simulink model "sampleModel264"  (R2021b)
settings: Solver=VariableStepAuto  StartTime=0.0  StopTime=10.0  RelTol=1e-3
undefined symbols (not defined in the file or in its folder): DiscIntNeverNeededParam
libraries: simulink x3, slpidlib x2
settings Model: Creator=user  LastModifiedBy=user

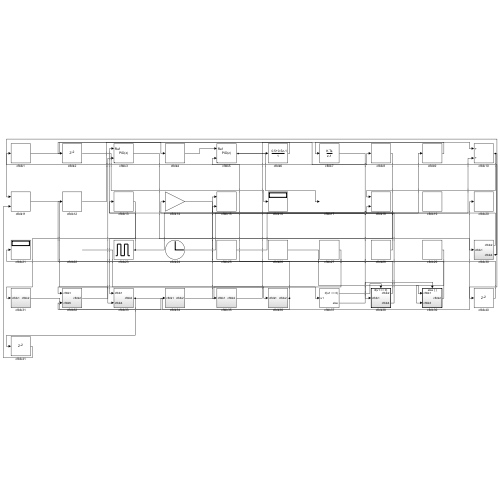
[thumbnail: Simulink's stored preview of the top-level diagram]
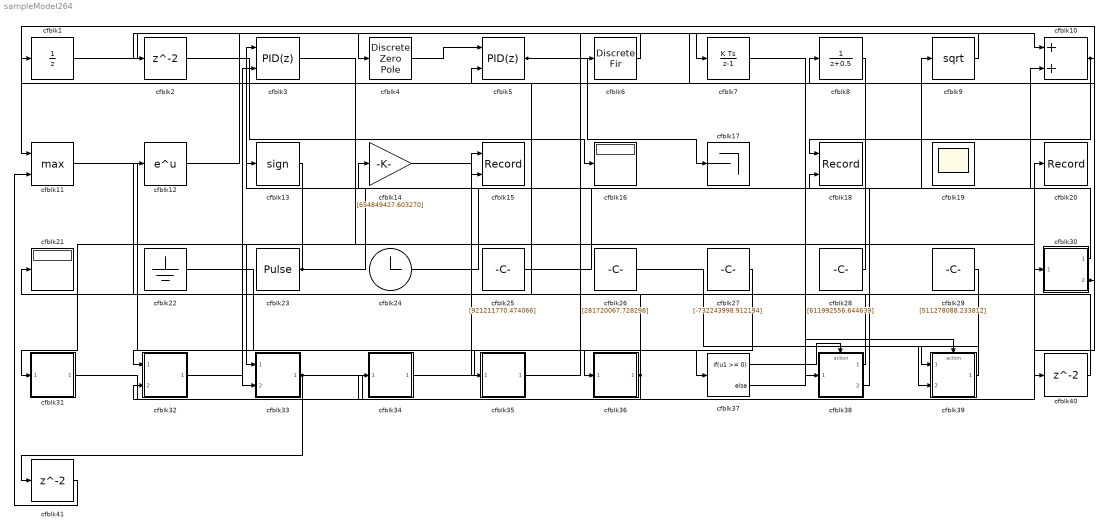
== system sampleModel264 ==
  cfblk1 : UnitDelay  HasFrameUpgradeWarning=on
  cfblk10 : Sum
  cfblk11 : MinMax  Function=max  Inputs=2
  cfblk12 : Math  SaturateOnIntegerOverflow=on
  cfblk13 : Signum
  cfblk14 : Gain  Gain=[654849427.603270]
  cfblk15 : Record  FileSettingsInternal="{\"entries\":[{\"content\":{\"excelSettings\":{\"content\":{},\"type\":\"Streamout.ExcelSettings\"}},\"type\":\"Streamout.FileSettingStorage\",\"uuid\":\"87b09053-a77a-4a9e-8bec-8608d5d060ef\"}],\"packageUris\":[\"http://schema.mathworks.com/mf0/streamout_blocks/R2020a\"],\"version\":\"1.0\"}"  Layout=[1 1]  SignalsInternal="{\"entries\":[{\"content\":{\"signals\":[{\"content\":{\"blockPath\":[\"sampleModel264/cfblk15\"],\"channel\":[],\"dimensions\":[1],\"domain\":\"sampleModel264/cfblk15\",\"lineColor\":\"#a2142f\",\"plots\":[1],\"port\":1,\"sid\":[\"\"],\"signalID\":10963,\"signalName\":\"cfblk38:1\"},\"type\":\"RecordBlkView.Signal\",\"uuid\":\"1c1d3461-8ecc-4c0c-aa7a-5d9b7c4e959a\"},{\"content\":{\"blockPath\":[\"sampleModel264/cfblk15\"],\"channel\":[],\"dimensions\":[1],\"domain\":\"sampleModel264/cfblk15\",\"lineColor\":\"#139fff\",\"plots\":[1],\"port\":2,\"sid\":[\"\"],\"signalID\":10967,\"signalName\":\"cfblk30:1\"},\"type\":\"RecordBlkView.Signal\",\"uuid\":\"7ac7cff1-7016-4733-9738-e051f763ac4b\"}]},\"type\":\"RecordBlkView.InputSignals\",\"uuid\":\"cdef2423-249f-4fef-a01c-88f3f527eae3\"}],\"packageUris\":[\"http://schema.mathworks.com/mf0/streamout_blocks/R2020a\"],\"version\":\"1.0\"}"  VisualizationBindings="{\"xyplotplugin\":{\"info\":[{\"series\":[{\"bindingParametersList\":[{\"parameter\":\"X-Axis\",\"signalID\":10963,\"signalName\":\"cfblk38:1\"},{\"parameter\":\"Y-Axis\",\"signalID\":10967,\"signalName\":\"cfblk30:1\"}],\"seriesID\":8609}],\"subplotID\":1}]}}"  CompatibilityTag=XY
  cfblk16 : Display
  cfblk17 : Terminator
  cfblk18 : Record  FileSettingsInternal="{\"entries\":[{\"content\":{\"excelSettings\":{\"content\":{},\"type\":\"Streamout.ExcelSettings\"}},\"type\":\"Streamout.FileSettingStorage\",\"uuid\":\"e408a021-66fe-4499-80ff-48ba78554e90\"}],\"packageUris\":[\"http://schema.mathworks.com/mf0/streamout_blocks/R2020a\"],\"version\":\"1.0\"}"  Layout=[1 1]  SignalsInternal="{\"entries\":[{\"content\":{\"signals\":[{\"content\":{\"blockPath\":[\"sampleModel264/cfblk18\"],\"channel\":[],\"dimensions\":[1],\"domain\":\"sampleModel264/cfblk18\",\"lineColor\":\"#a2142f\",\"plots\":[1],\"port\":1,\"sid\":[\"\"],\"signalID\":10971,\"signalName\":\"cfblk10\"},\"type\":\"RecordBlkView.Signal\",\"uuid\":\"3a710b1b-58d1-44e6-873a-359d775209f8\"},{\"content\":{\"blockPath\":[\"sampleModel264/cfblk18\"],\"channel\":[],\"dimensions\":[1],\"domain\":\"sampleModel264/cfblk18\",\"lineColor\":\"#139fff\",\"plots\":[1],\"port\":2,\"sid\":[\"\"],\"signalID\":10975,\"signalName\":\"cfblk25\"},\"type\":\"RecordBlkView.Signal\",\"uuid\":\"b2371862-496e-4d84-a68e-603eda18343e\"}]},\"type\":\"RecordBlkView.InputSignals\",\"uuid\":\"b556cba2-bf7e-48f4-b2b5-74105ca156f6\"}],\"packageUris\":[\"http://schema.mathworks.com/mf0/streamout_blocks/R2020a\"],\"version\":\"1.0\"}"  VisualizationBindings="{\"xyplotplugin\":{\"info\":[{\"series\":[{\"bindingParametersList\":[{\"parameter\":\"X-Axis\",\"signalID\":10971,\"signalName\":\"cfblk10\"},{\"parameter\":\"Y-Axis\",\"signalID\":10975,\"signalName\":\"cfblk25\"}],\"seriesID\":10129}],\"subplotID\":1}]}}"  CompatibilityTag=XY
  cfblk19 : Scope
      settings: Floating=on
  cfblk2 : Delay  SampleTime=1
  cfblk20 : Record  FileSettingsInternal="{\"entries\":[{\"content\":{\"excelSettings\":{\"content\":{},\"type\":\"Streamout.ExcelSettings\"}},\"type\":\"Streamout.FileSettingStorage\",\"uuid\":\"be7c116d-fe5e-441c-a5bb-7647be8af16f\"}],\"packageUris\":[\"http://schema.mathworks.com/mf0/streamout_blocks/R2020a\"],\"version\":\"1.0\"}"  SignalsInternal="{\"entries\":[{\"content\":{\"signals\":[{\"content\":{\"blockPath\":[\"sampleModel264/cfblk20\"],\"channel\":[],\"dimensions\":[1],\"domain\":\"sampleModel264/cfblk20\",\"lineColor\":\"#ff6929\",\"plots\":[1],\"port\":1,\"sid\":[\"\"],\"signalID\":10979,\"signalName\":\"cfblk33\"},\"type\":\"RecordBlkView.Signal\",\"uuid\":\"b8781fc3-0edb-411b-9528-19bbc625d2f5\"}]},\"type\":\"RecordBlkView.InputSignals\",\"uuid\":\"c04048e7-6647-4468-bb8a-5f250a700c8b\"}],\"packageUris\":[\"http://schema.mathworks.com/mf0/streamout_blocks/R2020a\"],\"version\":\"1.0\"}"  VisualizationBindings="{\"sparklinesplugin\":{\"info\":[{\"bindingParametersList\":[],\"subplotID\":1}]}}"
  cfblk21 : Display
  cfblk22 : Ground
  cfblk23 : DiscretePulseGenerator  PulseType=Time based  Amplitude=[-625805775.989914]  Period=[26020905.178933]  PulseWidth=5  PhaseDelay=[3.000000]
  cfblk24 : Clock
  cfblk25 : Constant  Value=[921211770.474066]  SampleTime=1
  cfblk26 : Constant  Value=[281720067.728298]  SampleTime=1
  cfblk27 : Constant  Value=[-732243998.912194]  SampleTime=1
  cfblk28 : Constant  Value=[611992556.644639]  SampleTime=1
  cfblk29 : Constant  Value=[511278088.233812]  SampleTime=1
  cfblk3 : slpidlib/PID Controller (2DOF)  Controller=PID  Form=Parallel  TimeDomain=Discrete-time  UseExternalTs=off  SampleTime=1  IntegratorMethod=Forward Euler  FilterMethod=Forward Euler  ControllerParametersSource=internal  P=1  I=1  D=0  UseFilter=on  N=100  b=1  c=1  TunerSelectOption=Transfer Function Based (PID Tuner App)  InitialConditionSource=internal  InitialConditionForIntegrator=0  InitialConditionForFilter=0  DifferentiatorICPrevScaledInput=0  ExternalReset=none  TrackingMode=off  Kt=1  LimitOutput=off  SatLimitsSource=internal  UpperSaturationLimit=inf  LowerSaturationLimit=-inf  LinearizeAsGain=off  AntiWindupMode=none  Kb=1  POutMin=[]  POutMax=[]  IOutMin=[]  IOutMax=[]  DOutMin=[]  DOutMax=[]  NOutMin=[]  NOutMax=[]  bOutMin=[]  bOutMax=[]  cOutMin=[]  cOutMax=[]  SumOutMin=[]  SumOutMax=[]  SaturationOutMin=[]  SaturationOutMax=[]  PParamMin=[]  PParamMax=[]  IParamMin=[]  IParamMax=[]  DParamMin=[]  DParamMax=[]  NParamMin=[]  NParamMax=[]  bParamMin=[]  bParamMax=[]  cParamMin=[]  cParamMax=[]  KbParamMin=[]  KbParamMax=[]  KtParamMin=[]  KtParamMax=[]  KbOutMin=[]  KbOutMax=[]  KtOutMin=[]  KtOutMax=[]  IntegratorOutMin=[]  IntegratorOutMax=[]  FilterOutMin=[]  FilterOutMax=[]  SumI1OutMin=[]  SumI1OutMax=[]  SumI2OutMin=[]  SumI2OutMax=[]  SumI3OutMin=[]  SumI3OutMax=[]  SumI4OutMin=[]  SumI4OutMax=[]  SumDOutMin=[]  SumDOutMax=[]  Sum1OutMin=[]  Sum1OutMax=[]  Sum2OutMin=[]  Sum2OutMax=[]  Sum3OutMin=[]  Sum3OutMax=[]  DifferentiatorOutMin=[]  DifferentiatorOutMax=[]  FilterDiffOutCoefMin=[]  FilterDiffOutCoefMax=[]  ReciprocalOutMin=[]  ReciprocalOutMax=[]  SumDenOutMin=[]  SumDenOutMax=[]  SumNumOutMin=[]  SumNumOutMax=[]  DivideOutMin=[]  DivideOutMax=[]  UdiffTsProdOutMin=[]  UdiffTsProdOutMax=[]  NTsProdOutMin=[]  NTsProdOutMax=[]  UintegralTsProdOutMin=[]  UintegralTsProdOutMax=[]  UngainTsProdOutMin=[]  UngainTsProdOutMax=[]  IntegratorContinuousStateAttributes=''  IntegratorStateMustResolveToSignalObject=off  IntegratorRTWStateStorageClass=Auto  FilterContinuousStateAttributes=''  FilterStateMustResolveToSignalObject=off  FilterRTWStateStorageClass=Auto  ParallelPVariant=InternalParameters  IdealPVariant=Disabled  IVariant=InternalParameters  DVariant=InternalParameters  bVariant=InternalParameters  cVariant=InternalParameters  IntegratorVariant=Discrete  SatVariant=Disabled  AWVariant=Passthrough  PCopyVariant=Disabled  TRVariant=Disabled  FdbkBlocksVariant=Forward  IdealPFdbkVariant=Disabled  SatFdbkVariant=Disabled  DerivativeFilterVariant=ForwardEulerFilter  NVariant=InternalParameters  NCopyVariant=Disabled  FilterICVariant=InternalICsFilter  IntegratorICVariant=InternalICs  ExternalResetVariant=Disabled  TRSumVariant=Passthrough  SumFdbkVariant=Disabled  SumVariant=Sum_PID  TsampFilterVariant=InternalTs  TsampNgainVariant=Passthrough  TsampIntegralVariant=Passthrough  ExternalSaturationOutDataTypeStr=Inherit: Same as second input
      settings: SourceProductBaseCode=SL
  cfblk30 : Subsystem
  cfblk31 : Subsystem
  cfblk32 : Subsystem
  cfblk33 : Subsystem
  cfblk34 : Subsystem
  cfblk35 : Subsystem
  cfblk36 : Subsystem
  cfblk37 : If  IfExpression=u1 >= 0  SampleTime=1
  cfblk38 : Subsystem  TreatAsAtomicUnit=on
  cfblk39 : Subsystem  TreatAsAtomicUnit=on
  cfblk4 : DiscreteZeroPole  Poles=[0 0.5]  Gain=1
  cfblk40 : Delay  SampleTime=1
  cfblk41 : Delay  SampleTime=1
  cfblk5 : slpidlib/PID Controller (2DOF)  Controller=PID  Form=Parallel  TimeDomain=Discrete-time  UseExternalTs=off  SampleTime=1  IntegratorMethod=Forward Euler  FilterMethod=Forward Euler  ControllerParametersSource=internal  P=1  I=1  D=0  UseFilter=on  N=100  b=1  c=1  TunerSelectOption=Transfer Function Based (PID Tuner App)  InitialConditionSource=internal  InitialConditionForIntegrator=0  InitialConditionForFilter=0  DifferentiatorICPrevScaledInput=0  ExternalReset=none  TrackingMode=off  Kt=1  LimitOutput=off  SatLimitsSource=internal  UpperSaturationLimit=inf  LowerSaturationLimit=-inf  LinearizeAsGain=off  AntiWindupMode=none  Kb=1  POutMin=[]  POutMax=[]  IOutMin=[]  IOutMax=[]  DOutMin=[]  DOutMax=[]  NOutMin=[]  NOutMax=[]  bOutMin=[]  bOutMax=[]  cOutMin=[]  cOutMax=[]  SumOutMin=[]  SumOutMax=[]  SaturationOutMin=[]  SaturationOutMax=[]  PParamMin=[]  PParamMax=[]  IParamMin=[]  IParamMax=[]  DParamMin=[]  DParamMax=[]  NParamMin=[]  NParamMax=[]  bParamMin=[]  bParamMax=[]  cParamMin=[]  cParamMax=[]  KbParamMin=[]  KbParamMax=[]  KtParamMin=[]  KtParamMax=[]  KbOutMin=[]  KbOutMax=[]  KtOutMin=[]  KtOutMax=[]  IntegratorOutMin=[]  IntegratorOutMax=[]  FilterOutMin=[]  FilterOutMax=[]  SumI1OutMin=[]  SumI1OutMax=[]  SumI2OutMin=[]  SumI2OutMax=[]  SumI3OutMin=[]  SumI3OutMax=[]  SumI4OutMin=[]  SumI4OutMax=[]  SumDOutMin=[]  SumDOutMax=[]  Sum1OutMin=[]  Sum1OutMax=[]  Sum2OutMin=[]  Sum2OutMax=[]  Sum3OutMin=[]  Sum3OutMax=[]  DifferentiatorOutMin=[]  DifferentiatorOutMax=[]  FilterDiffOutCoefMin=[]  FilterDiffOutCoefMax=[]  ReciprocalOutMin=[]  ReciprocalOutMax=[]  SumDenOutMin=[]  SumDenOutMax=[]  SumNumOutMin=[]  SumNumOutMax=[]  DivideOutMin=[]  DivideOutMax=[]  UdiffTsProdOutMin=[]  UdiffTsProdOutMax=[]  NTsProdOutMin=[]  NTsProdOutMax=[]  UintegralTsProdOutMin=[]  UintegralTsProdOutMax=[]  UngainTsProdOutMin=[]  UngainTsProdOutMax=[]  IntegratorContinuousStateAttributes=''  IntegratorStateMustResolveToSignalObject=off  IntegratorRTWStateStorageClass=Auto  FilterContinuousStateAttributes=''  FilterStateMustResolveToSignalObject=off  FilterRTWStateStorageClass=Auto  ParallelPVariant=InternalParameters  IdealPVariant=Disabled  IVariant=InternalParameters  DVariant=InternalParameters  bVariant=InternalParameters  cVariant=InternalParameters  IntegratorVariant=Discrete  SatVariant=Disabled  AWVariant=Passthrough  PCopyVariant=Disabled  TRVariant=Disabled  FdbkBlocksVariant=Forward  IdealPFdbkVariant=Disabled  SatFdbkVariant=Disabled  DerivativeFilterVariant=ForwardEulerFilter  NVariant=InternalParameters  NCopyVariant=Disabled  FilterICVariant=InternalICsFilter  IntegratorICVariant=InternalICs  ExternalResetVariant=Disabled  TRSumVariant=Passthrough  SumFdbkVariant=Disabled  SumVariant=Sum_PID  TsampFilterVariant=InternalTs  TsampNgainVariant=Passthrough  TsampIntegralVariant=Passthrough  ExternalSaturationOutDataTypeStr=Inherit: Same as second input
      settings: SourceProductBaseCode=SL
  cfblk6 : DiscreteFir  SampleTime=1
  cfblk7 : DiscreteIntegrator  ICPrevOutput=DiscIntNeverNeededParam  ICPrevScaledInput=DiscIntNeverNeededParam
  cfblk8 : DiscreteTransferFcn  SampleTime=1
  cfblk9 : Sqrt  SaturateOnIntegerOverflow=on
  wires:
  cfblk5/1 -> cfblk17/1, cfblk10/1
  cfblk23/1 -> cfblk3/1, cfblk10/2
  cfblk9/1 -> cfblk7/1
  cfblk12/1 -> cfblk8/1
  cfblk1/1 -> cfblk4/1
  cfblk2/1 -> cfblk16/1
  cfblk36/1(cfblk2) -> cfblk21/1, cfblk32/2(cfblk5)
  cfblk33/1(cfblk2) -> cfblk20/1, cfblk41/1
  cfblk34/1(cfblk2) -> cfblk37/1
  cfblk13/1 -> cfblk31/1(cfblk1)
  cfblk8/1 -> cfblk33/1(cfblk1)
  cfblk22/1 -> cfblk36/1(cfblk1)
  cfblk26/1 -> cfblk39/1(cfblk1)
  cfblk35/1(cfblk2) -> cfblk6/1
  cfblk31/1(cfblk2) -> cfblk34/1(cfblk1)
  cfblk32/1(cfblk2) -> cfblk3/2
  cfblk11/1 -> cfblk33/2(cfblk4)
  cfblk38/1(cfblk2) -> cfblk15/1
  cfblk28/1 -> cfblk13/1
  cfblk14/1 -> cfblk35/1(cfblk1)
  cfblk39/1(cfblk2) -> cfblk12/1
  cfblk3/1 -> cfblk30/1(cfblk1)
  cfblk29/1 -> cfblk39/2(cfblk3)
  cfblk38/2(cfblk4) -> cfblk14/1
  cfblk6/1 -> cfblk2/1
  cfblk24/1 -> cfblk9/1
  cfblk30/1(cfblk2) -> cfblk15/2
  cfblk30/2(cfblk4) -> cfblk11/1, cfblk1/1
  cfblk7/1 -> cfblk38/1(cfblk1)
  cfblk10/1 -> cfblk18/1, cfblk40/1
  cfblk4/1 -> cfblk5/1
  cfblk27/1 -> cfblk32/1(cfblk1)
  cfblk25/1 -> cfblk18/2
  cfblk37/1 -> cfblk38/Action
  cfblk37/2 -> cfblk39/Action
  cfblk40/1 -> cfblk5/2
  cfblk41/1 -> cfblk11/2

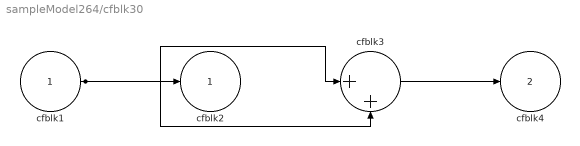
== system sampleModel264/cfblk30 ==
  cfblk1 : Inport
  cfblk3 : Sum  Inputs=|++
  cfblk2 : Outport
  cfblk4 : Outport  Port=2
  wires:
  cfblk3/1 -> cfblk4/1
  cfblk1/1 -> cfblk2/1, cfblk3/1, cfblk3/2

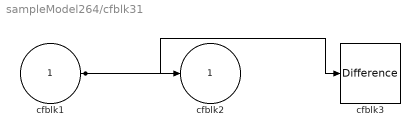
== system sampleModel264/cfblk31 ==
  cfblk1 : Inport
  cfblk3 : simulink/Discrete/Difference  ICPrevInput=0.0  OutMin=[]  OutMax=[]  OutDataTypeStr=Inherit: Inherit via back propagation  OutDataType=fixdt(1, 16)  OutScaling=2^-10  DoSatur=off
  cfblk2 : Outport
  wires:
  cfblk1/1 -> cfblk2/1, cfblk3/1

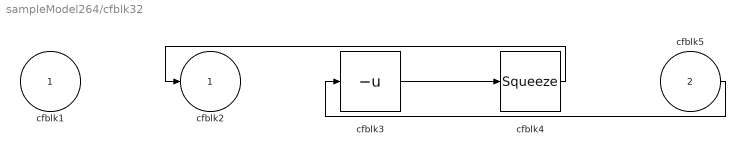
== system sampleModel264/cfblk32 ==
  cfblk1 : Inport
  cfblk5 : Inport  Port=2
  cfblk3 : UnaryMinus
  cfblk4 : Squeeze
  cfblk2 : Outport
  wires:
  cfblk4/1 -> cfblk2/1
  cfblk5/1 -> cfblk3/1
  cfblk3/1 -> cfblk4/1

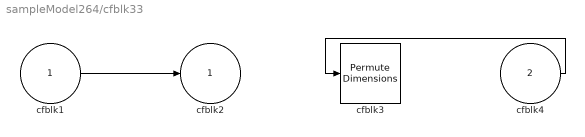
== system sampleModel264/cfblk33 ==
  cfblk1 : Inport
  cfblk4 : Inport  Port=2
  cfblk3 : PermuteDimensions
  cfblk2 : Outport
  wires:
  cfblk4/1 -> cfblk3/1
  cfblk1/1 -> cfblk2/1

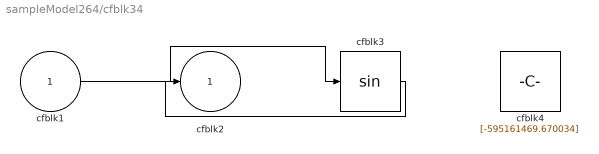
== system sampleModel264/cfblk34 ==
  cfblk1 : Inport
  cfblk3 : Trigonometry
  cfblk4 : Constant  Value=[-595161469.670034]  SampleTime=1
  cfblk2 : Outport
  wires:
  cfblk1/1 -> cfblk3/1
  cfblk3/1 -> cfblk2/1

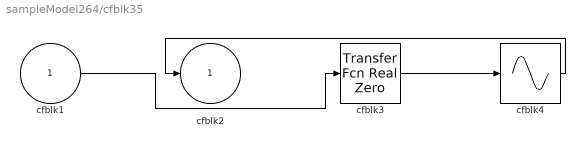
== system sampleModel264/cfblk35 ==
  cfblk1 : Inport
  cfblk3 : simulink/Discrete/Transfer Fcn Real Zero  ZeroZ=0.75  ICPrevInput=0.0  DoSatur=off
      settings: SourceProductBaseCode=SL
  cfblk4 : Sin  TimeSource=Use external signal  SampleTime=0
  cfblk2 : Outport
  wires:
  cfblk3/1 -> cfblk4/1
  cfblk4/1 -> cfblk2/1
  cfblk1/1 -> cfblk3/1

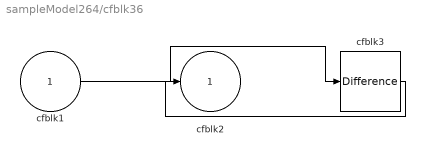
== system sampleModel264/cfblk36 ==
  cfblk1 : Inport
  cfblk3 : simulink/Discrete/Difference  ICPrevInput=0.0  OutMin=[]  OutMax=[]  OutDataTypeStr=Inherit: Inherit via back propagation  OutDataType=fixdt(1, 16)  OutScaling=2^-10  DoSatur=off
  cfblk2 : Outport
  wires:
  cfblk1/1 -> cfblk3/1
  cfblk3/1 -> cfblk2/1

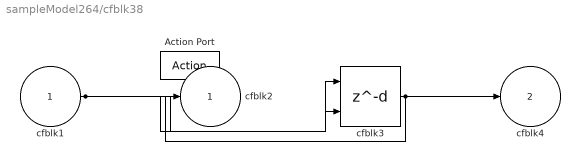
== system sampleModel264/cfblk38 ==
  cfblk1 : Inport
  Action Port : ActionPort  ActionPortLabel=if(u1 >= 0)
  cfblk3 : Delay  DelayLengthSource=Input port
      settings: InputPortMap=u0,p1
  cfblk2 : Outport
  cfblk4 : Outport  Port=2
  wires:
  cfblk1/1 -> cfblk3/1, cfblk3/2
  cfblk3/1 -> cfblk2/1, cfblk4/1

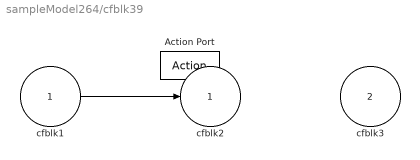
== system sampleModel264/cfblk39 ==
  cfblk1 : Inport
  cfblk3 : Inport  Port=2
  Action Port : ActionPort  ActionPortLabel=else
  cfblk2 : Outport
  wires:
  cfblk1/1 -> cfblk2/1
